simulink model "balancer"  (R2012b)
settings: Solver=ode45  StartTime=0.0  StopTime=10  RelTol=1e-3
settings Model: Creator=spin7ion  LastModifiedBy=spin7ion

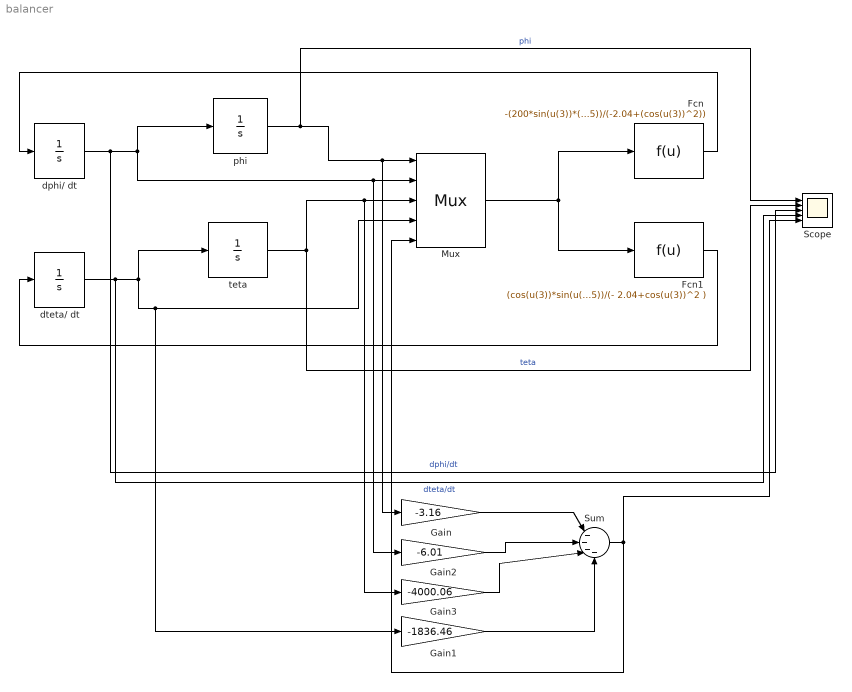
== system balancer ==
  Fcn : Fcn  Expr=-(200*sin(u(3))*(u(4)^2)-980*cos(u(3))*sin(u(3))+20000*u(5))/(-2.04+(cos(u(3))^2))
  Fcn1 : Fcn  Expr=(cos(u(3))*sin(u(3))*u(4)^2-9.996*sin(u(3))+100*cos(u(3))*u(5))/(- 2.04+cos(u(3))^2 )
  Gain : Gain  Gain=-3.16
  Gain1 : Gain  Gain=-1836.46
  Gain2 : Gain  Gain=-6.01
  Gain3 : Gain  Gain=-4000.06
  Mux : Mux  Inputs=5
      settings: DisplayOption=signals
  Scope : Scope  NumInputPorts=5
      settings: YMin=0~-0.15~-200~-2~-1500  YMax=50~0.1~500~1~1000  MaxDataPoints=1000000000
  Sum : Sum  Inputs=|----
  dphi/ dt : Integrator
  dteta/ dt : Integrator
  phi : Integrator
  teta : Integrator  InitialCondition=0.1
  wires:
  dphi/ dt/1 -> phi/1, Gain2/1, Mux/2, Scope/3  "dphi/dt"
  teta/1 -> Mux/3, Gain3/1, Scope/2  "teta"
  dteta/ dt/1 -> teta/1, Gain1/1, Mux/4, Scope/4  "dteta/dt"
  phi/1 -> Gain/1, Mux/1, Scope/1  "phi"
  Mux/1 -> Fcn1/1, Fcn/1
  Fcn/1 -> dphi/ dt/1
  Gain/1 -> Sum/1
  Gain2/1 -> Sum/2
  Gain3/1 -> Sum/3
  Gain1/1 -> Sum/4
  Fcn1/1 -> dteta/ dt/1
  Sum/1 -> Mux/5, Scope/5
